simulink model "Exercise_3_1"  (R2022a)
settings: Solver=VariableStepAuto  StartTime=0.0  StopTime=30  RelTol=1e-3
libraries: simulink_extras x6, m3dof_library x6, simulink x2
settings Model: Creator=s9203  LastModifiedBy=s9203

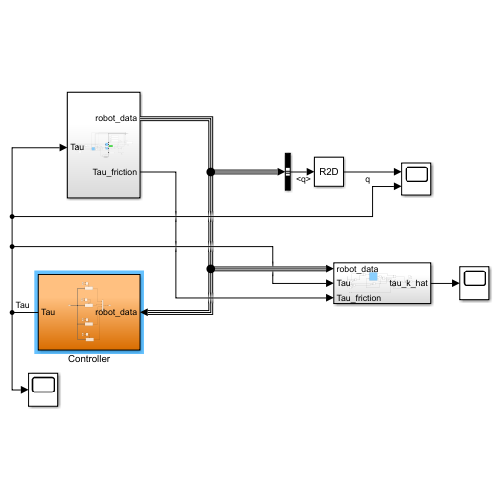
[thumbnail: Simulink's stored preview of the top-level diagram]
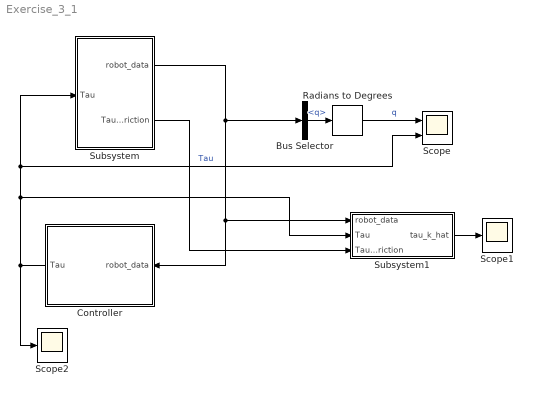
== system Exercise_3_1 ==
  Bus Selector : BusSelector  OutputSignals=q
  Controller : Subsystem
  Radians to Degrees : simulink_extras/Transformations/Radians to Degrees
  Scope : Scope  NumInputPorts=2
  Scope1 : Scope
  Scope2 : Scope
  Subsystem : Subsystem
  Subsystem1 : Subsystem
  wires:
  Subsystem/1(robot_data) -> Bus Selector/1, Controller/1(robot_data), Subsystem1/1(robot_data)
  Controller/1(Tau) -> Scope/2, Subsystem/1(Tau), Subsystem1/2(Tau), Scope2/1  "Tau"
  Bus Selector/1 -> Radians to Degrees/1  "<q>"
  Radians to Degrees/1 -> Scope/1  "q"
  Subsystem1/1(tau_k_hat) -> Scope1/1
  Subsystem/2(Tau_friction) -> Subsystem1/3(Tau_friction)

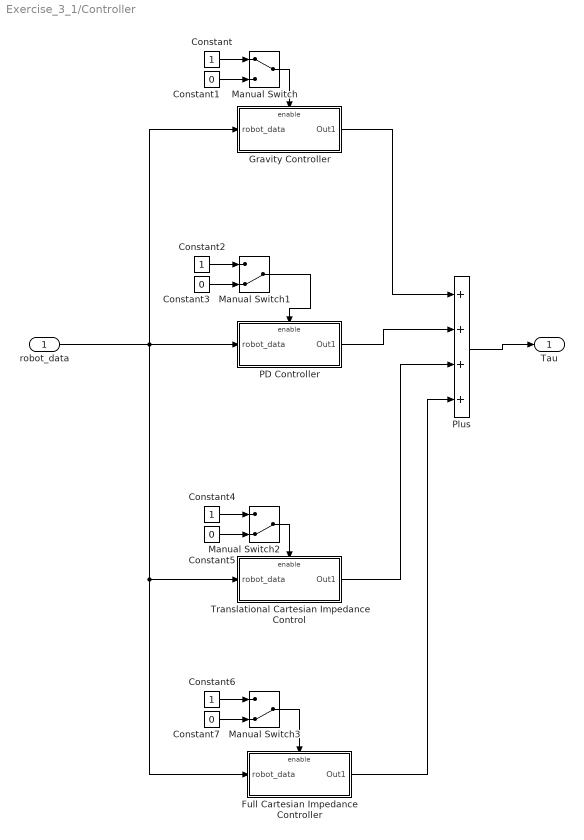
== system Exercise_3_1/Controller ==
  robot_data : Inport
  Constant{,2,4,6} (4 alike) : Constant
  Constant{1,3,5,7} (4 alike) : Constant  Value=0
  Full Cartesian Impedance Controller : Subsystem  TreatAsAtomicUnit=on
  Gravity Controller : Subsystem  TreatAsAtomicUnit=on
  Manual Switch : ManualSwitch
  Manual Switch1 : ManualSwitch  CurrentSetting=0
  Manual Switch2 : ManualSwitch  CurrentSetting=0
  Manual Switch3 : ManualSwitch  CurrentSetting=0
  "PD Controller " : Subsystem  TreatAsAtomicUnit=on
  Plus : Sum  Inputs=++++
  Translational Cartesian Impedance Control : Subsystem  TreatAsAtomicUnit=on
  Tau : Outport
  wires:
  robot_data/1 -> Full Cartesian Impedance Controller/1(robot_data), Translational Cartesian Impedance Control/1(robot_data), "PD Controller "/1(robot_data), Gravity Controller/1(robot_data)
  Gravity Controller/1(Out1) -> Plus/1
  "PD Controller "/1(Out1) -> Plus/2
  Translational Cartesian Impedance Control/1(Out1) -> Plus/3
  Plus/1 -> Tau/1
  Constant/1 -> Manual Switch/1
  Constant1/1 -> Manual Switch/2
  Manual Switch/1 -> Gravity Controller/Enable
  Constant3/1 -> Manual Switch1/2
  Constant2/1 -> Manual Switch1/1
  Constant4/1 -> Manual Switch2/1
  Constant5/1 -> Manual Switch2/2
  Manual Switch2/1 -> Translational Cartesian Impedance Control/Enable
  Manual Switch1/1 -> "PD Controller "/Enable
  Manual Switch3/1 -> Full Cartesian Impedance Controller/Enable
  Constant7/1 -> Manual Switch3/2
  Constant6/1 -> Manual Switch3/1
  Full Cartesian Impedance Controller/1(Out1) -> Plus/4

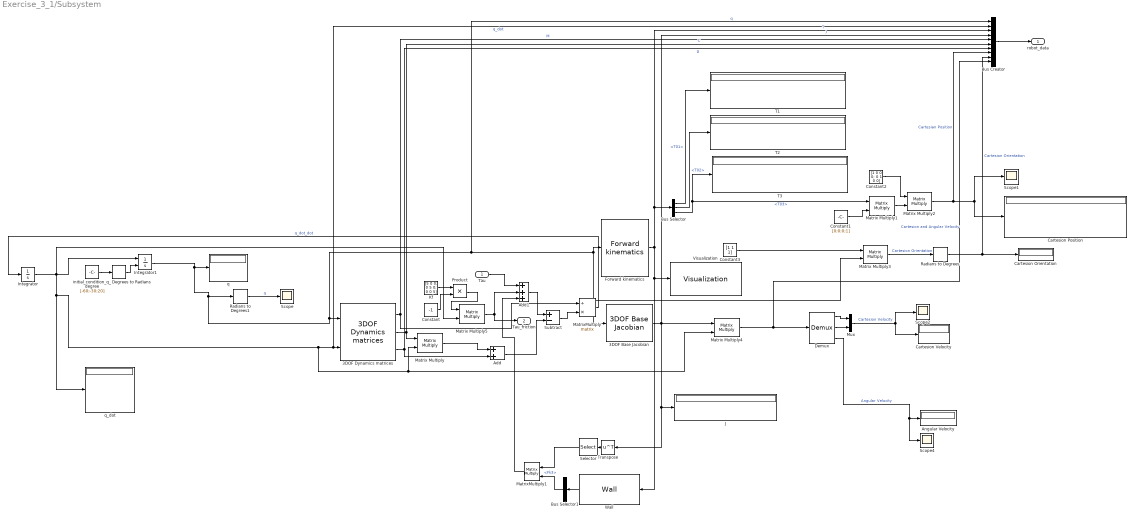
== system Exercise_3_1/Subsystem ==
  Tau : Inport
  3DOF Base Jacobian : m3dof_library/3DOF Base Jacobian  a1=l1  a2=l2  a3=l3
  3DOF Dynamics matrices : m3dof_library/3DOF Dynamics matrices  m1=m1  mX1=mx1  ZZ1=I1  m2=m2  mX2=mx2  ZZ2=I2  m3=m3  mX3=mx3  ZZ3=I3  a1=l1  a2=l2  a3=l3  eg=eg
  Add : Sum
  Add1 : Sum  Inputs=+++
  Angular Velocity : Display
  Bus Creator : BusCreator  Inputs=10
  Bus Selector : BusSelector  OutputSignals=T01,T02,T03
  Bus Selector1 : BusSelector  OutputSignals=Fk3
  Cartesion Orientation : Display
  Cartesion Position : Display
  Cartesion Velocity : Display
  Constant : Constant  Value=-1
  Constant1 : Constant  Value=[0;0;0;1]
  Constant2 : Constant  Value=[1 0 0 0; 0 1 0 0]
  Constant3 : Constant  Value=[1 1 1]  VectorParams1D=off
  Degrees to Radians : simulink_extras/Transformations/Degrees to Radians
  Demux : Demux  Outputs=3
      settings: DisplayOption=none
  Forward kinematics : m3dof_library/Forward kinematics  a1=l1  a2=l2  a3=l3  alpha=0
  Integrator : Integrator
  Integrator1 : Integrator  InitialConditionSource=external
  J : Display
  Kf : Constant  Value=[5 0 0; 0 5 0; 0 0 5]
  Matrix Multiply{,1..5} (6 alike) : Product  Multiplication=Matrix(*)
  MatrixMultiply : Product  Inputs=/*  Multiplication=Matrix(*)
  MatrixMultiply1 : Product  Multiplication=Matrix(*)
  Mux : Mux  Inputs=2
  Product : Product
  Radians to Degrees : simulink_extras/Transformations/Radians to Degrees
  Radians to Degrees1 : simulink_extras/Transformations/Radians to Degrees
  Scope{,1..2,4} (4 alike) : Scope
  Selector : Selector  NumberOfDimensions=2  InputPortWidth=3  IndexOptions=Index vector (dialog),Index vector (dialog)  Indices=[1 2 3],[1 2]  OutputSizes=1,1
  Subtract : Sum  Inputs=+-
  T1 : Display
  T2 : Display
  T3 : Display
  Transpose : Math  Operator=transpose
  Visualization : m3dof_library/Visualization  Ts0=1/16  al=1  a1=l1  a2=l2  a3=l3  alpha=0  eg=eg  tl=50
  Wall : m3dof_library/Wall  x0=[1.2 0]  w=[-1 0]
  "initial_condition_q_degree " : Constant  Value=[-60;-30;20]
  q : Display
  q_dot : Display
  robot_data : Outport
  Tau_friction : Outport  Port=2
  wires:
  Integrator/1 -> Matrix Multiply4/2, Matrix Multiply/2, Bus Creator/2, 3DOF Dynamics matrices/2, q_dot/1, Integrator1/1, Matrix Multiply5/2  "q_dot"
  Demux/3 -> Scope4/1, Angular Velocity/1  "Angular Velocity"
  3DOF Dynamics matrices/1 -> Bus Creator/5, MatrixMultiply/1  "M"
  Forward kinematics/1 -> Visualization/1, Wall/1, Bus Selector/1, Bus Creator/3  "T"
  Demux/1 -> Mux/1
  3DOF Base Jacobian/1 -> Transpose/1, J/1, Matrix Multiply4/1, Bus Creator/4  "J"
  Add1/1 -> Subtract/1
  Degrees to Radians/1 -> Integrator1/2
  Demux/2 -> Mux/2
  Matrix Multiply2/1 -> Bus Creator/8, Cartesion Position/1, Scope1/1  "Cartesian Position"
  3DOF Dynamics matrices/3 -> Bus Creator/7, Add/2  "g"
  Mux/1 -> Cartesion Velocity/1, Scope2/1  "Cartesion Velocity"
  Matrix Multiply/1 -> Add/1
  Radians to Degrees/1 -> Cartesion Orientation/1, Bus Creator/9  "Cartesion Orientation"
  MatrixMultiply/1 -> Integrator/1  "q_dot_dot"
  3DOF Dynamics matrices/2 -> Bus Creator/6, Matrix Multiply/1  "C"
  Constant/1 -> Product/2
  Matrix Multiply5/1 -> Add1/2, Tau_friction/1
  Bus Selector/3 -> Matrix Multiply1/1, T3/1  "<T03>"
  "initial_condition_q_degree "/1 -> Degrees to Radians/1
  Bus Selector/2 -> T2/1  "<T02>"
  Constant1/1 -> Matrix Multiply1/2
  Matrix Multiply3/1 -> Radians to Degrees/1  "Cartesion Orientation"
  Constant3/1 -> Matrix Multiply3/1
  Bus Selector/1 -> T1/1  "<T01>"
  Constant2/1 -> Matrix Multiply2/1
  Add/1 -> Subtract/2
  Matrix Multiply1/1 -> Matrix Multiply2/2
  Matrix Multiply4/1 -> Bus Creator/10, Demux/1  "Cartesion and Angular Velocity"
  Bus Creator/1 -> robot_data/1
  Kf/1 -> Product/1
  Product/1 -> Matrix Multiply5/1
  Integrator1/1 -> Radians to Degrees1/1, Bus Creator/1, 3DOF Base Jacobian/1, Matrix Multiply3/2, Forward kinematics/1, 3DOF Dynamics matrices/1, q/1  "q"
  Wall/1 -> Bus Selector1/1
  Transpose/1 -> Selector/1
  Selector/1 -> MatrixMultiply1/1
  Bus Selector1/1 -> MatrixMultiply1/2  "<Fk3>"
  MatrixMultiply1/1 -> Add1/3
  Subtract/1 -> MatrixMultiply/2
  Radians to Degrees1/1 -> Scope/1  "q"
  Tau/1 -> Add1/1

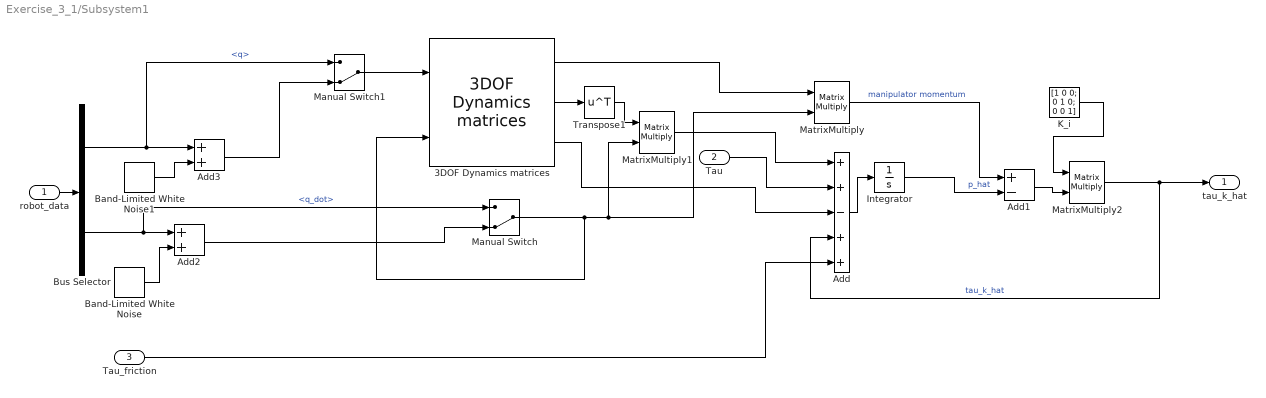
== system Exercise_3_1/Subsystem1 ==
  robot_data : Inport
  Tau : Inport  Port=2
  Tau_friction : Inport  Port=3
  3DOF Dynamics matrices : m3dof_library/3DOF Dynamics matrices  m1=m1  mX1=mx1  ZZ1=I1  m2=m2  mX2=mx2  ZZ2=I2  m3=m3  mX3=mx3  ZZ3=I3  a1=l1  a2=l2  a3=l3  eg=eg
  Add : Sum  Inputs=++-++
  Add1 : Sum  Inputs=+-
  Add2 : Sum
  Add3 : Sum
  Band-Limited White Noise : simulink/Sources/Band-Limited White Noise  Cov=[0.0001]  Ts=0.1  seed=[23341]
  Band-Limited White Noise1 : simulink/Sources/Band-Limited White Noise  Cov=[0.0001]  Ts=0.1  seed=[23341]
  Bus Selector : BusSelector  OutputSignals=q,q_dot
  Integrator : Integrator
  K_i : Constant  Value=[1 0 0; 0 1 0; 0 0 1]
  Manual Switch : ManualSwitch  CurrentSetting=0
  Manual Switch1 : ManualSwitch  CurrentSetting=0
  MatrixMultiply : Product  Multiplication=Matrix(*)
  MatrixMultiply1 : Product  Multiplication=Matrix(*)
  MatrixMultiply2 : Product  Multiplication=Matrix(*)
  Transpose1 : Math  Operator=transpose
  tau_k_hat : Outport
  wires:
  robot_data/1 -> Bus Selector/1
  3DOF Dynamics matrices/1 -> MatrixMultiply/1
  Manual Switch/1 -> MatrixMultiply/2, MatrixMultiply1/2, 3DOF Dynamics matrices/2
  3DOF Dynamics matrices/2 -> Transpose1/1
  Transpose1/1 -> MatrixMultiply1/1
  3DOF Dynamics matrices/3 -> Add/3
  Add/1 -> Integrator/1
  MatrixMultiply/1 -> Add1/1  "manipulator momentum"
  Integrator/1 -> Add1/2  "p_hat"
  Add1/1 -> MatrixMultiply2/2
  K_i/1 -> MatrixMultiply2/1
  MatrixMultiply2/1 -> Add/4, tau_k_hat/1  "tau_k_hat"
  Bus Selector/2 -> Manual Switch/1, Add2/1  "<q_dot>"
  Add2/1 -> Manual Switch/2
  Manual Switch1/1 -> 3DOF Dynamics matrices/1
  Bus Selector/1 -> Manual Switch1/1, Add3/1  "<q>"
  Add3/1 -> Manual Switch1/2
  Band-Limited White Noise1/1 -> Add3/2
  Band-Limited White Noise/1 -> Add2/2
  Tau/1 -> Add/2
  MatrixMultiply1/1 -> Add/1
  Tau_friction/1 -> Add/5

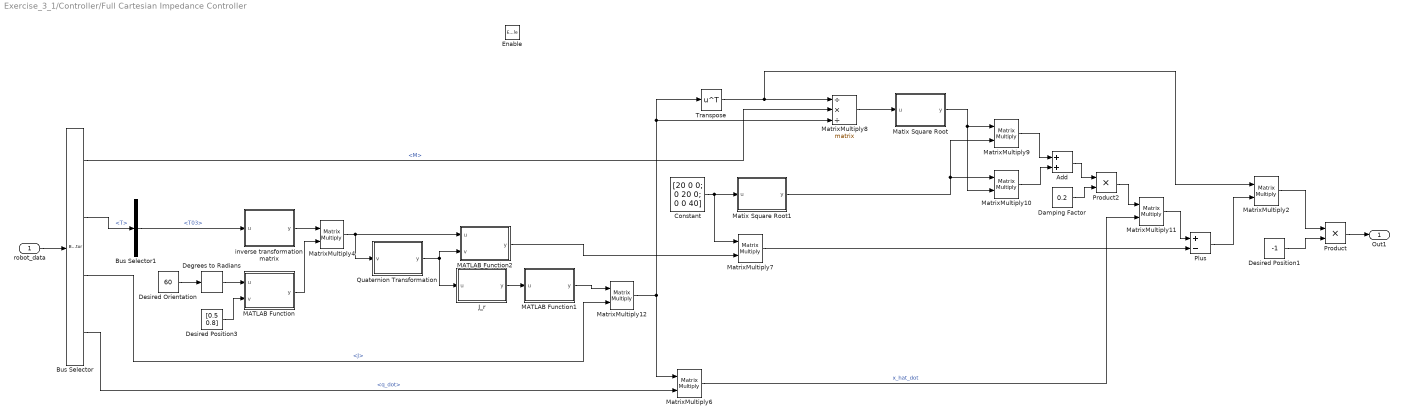
== system Exercise_3_1/Controller/Full Cartesian Impedance Controller ==
  robot_data : Inport
  Enable : EnablePort
  Add : Sum
  Bus Selector : BusSelector  OutputSignals=M,T,J,q_dot
  Bus Selector1 : BusSelector  OutputSignals=T03
  Constant : Constant  Value=[20 0 0; 0 20 0; 0 0 40]  VectorParams1D=off
  Damping Factor : Constant  Value=0.2
  Degrees to Radians : simulink_extras/Transformations/Degrees to Radians
  Desired Orientation : Constant  Value=60
  Desired Position1 : Constant  Value=-1
  Desired Position3 : Constant  Value=[0.5 0.8]  VectorParams1D=off
  J_r : MATLAB Function  TreatAsAtomicUnit=on
  MATLAB Function : MATLAB Function  TreatAsAtomicUnit=on
  MATLAB Function1 : MATLAB Function  TreatAsAtomicUnit=on
  MATLAB Function2 : MATLAB Function  TreatAsAtomicUnit=on
  Matix Square Root : MATLAB Function  TreatAsAtomicUnit=on
  Matix Square Root1 : MATLAB Function  TreatAsAtomicUnit=on
  MatrixMultiply{2,4,6..7,9..12} (8 alike) : Product  Multiplication=Matrix(*)
  MatrixMultiply8 : Product  Inputs=/*/  Multiplication=Matrix(*)
  Plus : Sum  Inputs=+-
  Product : Product
  Product2 : Product
  Quaternion Transformation : MATLAB Function  TreatAsAtomicUnit=on
  Transpose : Math  Operator=transpose
  inverse transformation matrix : MATLAB Function  TreatAsAtomicUnit=on
  Out1 : Outport
  wires:
  Transpose/1 -> MatrixMultiply2/1, MatrixMultiply8/1
  Desired Position1/1 -> Product/2
  MatrixMultiply2/1 -> Product/1
  Bus Selector/3 -> MatrixMultiply12/2  "<J>"
  Desired Position3/1 -> MATLAB Function/2(v)
  robot_data/1 -> Bus Selector/1
  Bus Selector/2 -> Bus Selector1/1  "<T>"
  Bus Selector1/1 -> inverse transformation matrix/1(u)  "<T03>"
  J_r/1(y) -> MATLAB Function1/1(u)
  Desired Orientation/1 -> Degrees to Radians/1
  Degrees to Radians/1 -> MATLAB Function/1(u)
  Bus Selector/4 -> MatrixMultiply6/2  "<q_dot>"
  MATLAB Function1/1(y) -> MatrixMultiply12/1
  MatrixMultiply6/1 -> MatrixMultiply11/2  "x_hat_dot"
  Quaternion Transformation/1(y) -> J_r/1(u), MATLAB Function2/2(v)
  Constant/1 -> MatrixMultiply7/1, Matix Square Root1/1(u)
  Bus Selector/1 -> MatrixMultiply8/2  "<M>"
  MatrixMultiply8/1 -> Matix Square Root/1(u)
  Matix Square Root/1(y) -> MatrixMultiply10/2, MatrixMultiply9/1
  Matix Square Root1/1(y) -> MatrixMultiply9/2, MatrixMultiply10/1
  MatrixMultiply9/1 -> Add/1
  MatrixMultiply10/1 -> Add/2
  Add/1 -> Product2/1
  Damping Factor/1 -> Product2/2
  Product2/1 -> MatrixMultiply11/1
  MatrixMultiply12/1 -> MatrixMultiply8/3, Transpose/1, MatrixMultiply6/1
  MATLAB Function/1(y) -> MatrixMultiply4/2
  inverse transformation matrix/1(y) -> MatrixMultiply4/1
  MatrixMultiply4/1 -> Quaternion Transformation/1(v), MATLAB Function2/1(u)
  Product/1 -> Out1/1
  MatrixMultiply7/1 -> Plus/2
  MatrixMultiply11/1 -> Plus/1
  Plus/1 -> MatrixMultiply2/2
  MATLAB Function2/1(y) -> MatrixMultiply7/2

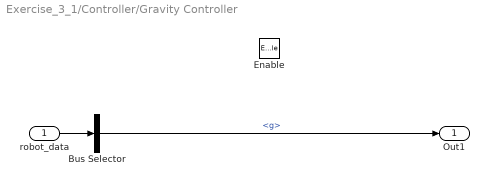
== system Exercise_3_1/Controller/Gravity Controller ==
  robot_data : Inport
  Enable : EnablePort
  Bus Selector : BusSelector  OutputSignals=g
  Out1 : Outport
  wires:
  robot_data/1 -> Bus Selector/1
  Bus Selector/1 -> Out1/1  "<g>"

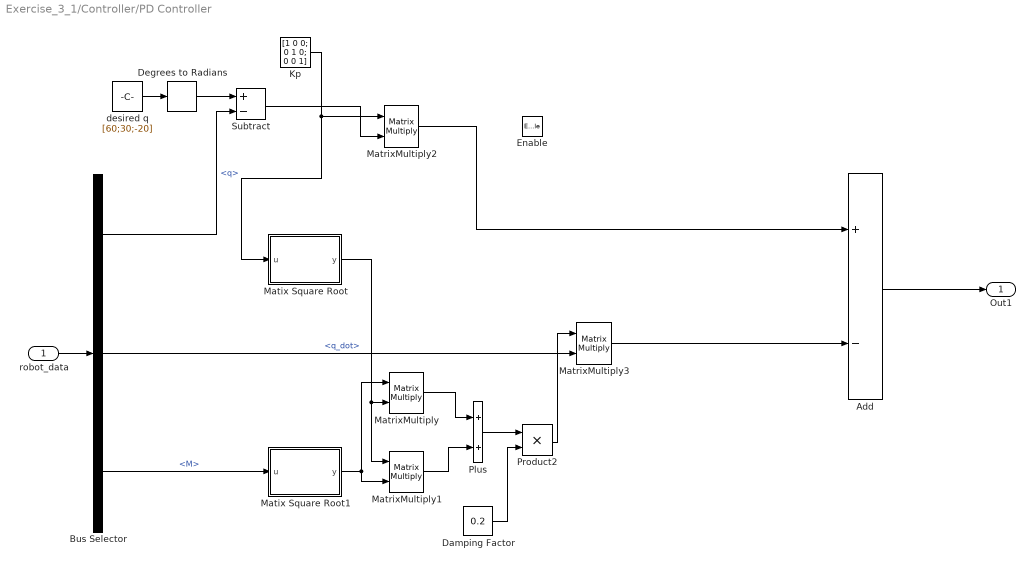
== system Exercise_3_1/Controller/PD Controller  ==
  robot_data : Inport
  Enable : EnablePort
  Add : Sum  Inputs=+-
  Bus Selector : BusSelector  OutputSignals=q,q_dot,M
  Damping Factor : Constant  Value=0.2
  Degrees to Radians : simulink_extras/Transformations/Degrees to Radians
  Kp : Constant  Value=[1 0 0; 0 1 0; 0 0 1]
  Matix Square Root : MATLAB Function  TreatAsAtomicUnit=on
  Matix Square Root1 : MATLAB Function  TreatAsAtomicUnit=on
  MatrixMultiply{,1..3} (4 alike) : Product  Multiplication=Matrix(*)
  Plus : Sum
  Product2 : Product
  Subtract : Sum  Inputs=+-
  desired q : Constant  Value=[60;30;-20]
  Out1 : Outport
  wires:
  Add/1 -> Out1/1
  desired q/1 -> Degrees to Radians/1
  robot_data/1 -> Bus Selector/1
  Degrees to Radians/1 -> Subtract/1
  Bus Selector/1 -> Subtract/2  "<q>"
  Subtract/1 -> MatrixMultiply2/2
  Kp/1 -> Matix Square Root/1(u), MatrixMultiply2/1
  MatrixMultiply2/1 -> Add/1
  MatrixMultiply3/1 -> Add/2
  Bus Selector/2 -> MatrixMultiply3/2  "<q_dot>"
  Bus Selector/3 -> Matix Square Root1/1(u)  "<M>"
  Matix Square Root1/1(y) -> MatrixMultiply1/2, MatrixMultiply/1
  Matix Square Root/1(y) -> MatrixMultiply1/1, MatrixMultiply/2
  MatrixMultiply/1 -> Plus/1
  MatrixMultiply1/1 -> Plus/2
  Plus/1 -> Product2/1
  Damping Factor/1 -> Product2/2
  Product2/1 -> MatrixMultiply3/1

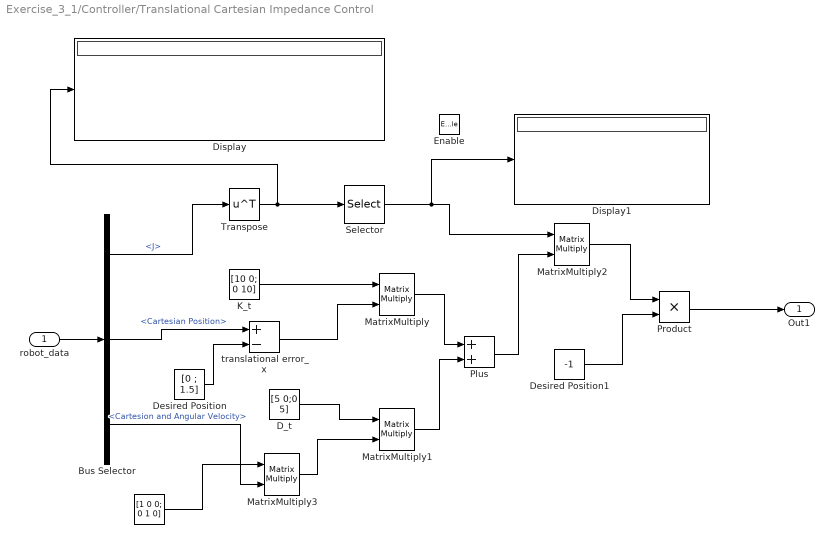
== system Exercise_3_1/Controller/Translational Cartesian Impedance Control ==
  robot_data : Inport
  Enable : EnablePort
  " " : Constant  Value=[1 0 0; 0 1 0]
  Bus Selector : BusSelector  OutputSignals=J,Cartesian Position,Cartesion and Angular Velocity
  D_t : Constant  Value=[5 0;0 5]
  Desired Position : Constant  Value=[0 ; 1.5]
  Desired Position1 : Constant  Value=-1
  Display : Display
  Display1 : Display
  K_t : Constant  Value=[10 0; 0 10]
  MatrixMultiply{,1..3} (4 alike) : Product  Multiplication=Matrix(*)
  Plus : Sum
  Product : Product
  Selector : Selector  NumberOfDimensions=2  InputPortWidth=3  IndexOptions=Index vector (dialog),Index vector (dialog)  Indices=[1 2 3],[1 2]  OutputSizes=1,1
  Transpose : Math  Operator=transpose
  translational error_x : Sum  Inputs=+-
  Out1 : Outport
  wires:
  robot_data/1 -> Bus Selector/1
  Desired Position/1 -> translational error_x/2
  Bus Selector/2 -> translational error_x/1  "<Cartesian Position>"
  K_t/1 -> MatrixMultiply/1
  translational error_x/1 -> MatrixMultiply/2
  D_t/1 -> MatrixMultiply1/1
  Bus Selector/1 -> Transpose/1  "<J>"
  MatrixMultiply/1 -> Plus/1
  MatrixMultiply1/1 -> Plus/2
  Plus/1 -> MatrixMultiply2/2
  MatrixMultiply2/1 -> Product/1
  Desired Position1/1 -> Product/2
  Product/1 -> Out1/1
  " "/1 -> MatrixMultiply3/1
  Bus Selector/3 -> MatrixMultiply3/2  "<Cartesion and Angular Velocity>"
  MatrixMultiply3/1 -> MatrixMultiply1/2
  Transpose/1 -> Display/1, Selector/1
  Selector/1 -> Display1/1, MatrixMultiply2/1

== matlab function Exercise_3_1/Controller/PD Controller /Matix Square Root1 ==
  data: u input; y output
function y = fcn(u)

y = real(sqrtm(u));

== matlab function Exercise_3_1/Controller/PD Controller /Matix Square Root ==
  data: u input; y output
function y = fcn(u)

y = real(sqrtm(u));

== matlab function Exercise_3_1/Controller/Full Cartesian Impedance Controller/J_r ==
  data: u input; y output
function y = fcn(u)
eta= u(1,1);
diag_eta = eta*[1 0 0; 0 1 0; 0 0 1];

epsilon = [-u(2,1) -u(3,1) -u(4,1)]';
skew_epsilon = [0 -epsilon(3) epsilon(2) ; epsilon(3) 0 -epsilon(1) ; -epsilon(2) epsilon(1) 0 ];

y = skew_epsilon + diag_eta;

== matlab function Exercise_3_1/Controller/Full Cartesian Impedance Controller/Quaternion Transformation ==
  data: v input; y output
function y = fcn(v)
u = v(1:3,1:3);

eta = 0.5*sqrt([1 1 1]*(diag(u).^2)+1);

epsilon_1 = (u(3,2)-u(2,3))/(4*eta);
epsilon_2 = (u(1,3)-u(3,1))/(4*eta);
epsilon_3 = (u(2,1)-u(1,2))/(4*eta);

y = [eta ; epsilon_1; epsilon_2; epsilon_3];

== matlab function Exercise_3_1/Controller/Full Cartesian Impedance Controller/MATLAB Function ==
  data: u input; y output; v input
function y = fcn(u,v)
Transformation_matrix = [cos(u) -sin(u) 0 v(1); sin(u) cos(u) 0 v(2); 0 0 1 0; 0 0 0 1];

y = Transformation_matrix;

== matlab function Exercise_3_1/Controller/Full Cartesian Impedance Controller/MATLAB Function1 ==
  data: u input; y output
function y = fcn(u)


y = [1 0 0; 0 1 0; 0 0 u(3,3)];

== matlab function Exercise_3_1/Controller/Full Cartesian Impedance Controller/Matix Square Root ==
  data: u input; y output
function y = fcn(u)

y = real(sqrtm(u));

== matlab function Exercise_3_1/Controller/Full Cartesian Impedance Controller/Matix Square Root1 ==
  data: u input; y output
function y = fcn(u)

y = real(sqrtm(u));

== matlab function Exercise_3_1/Controller/Full Cartesian Impedance Controller/inverse transformation matrix ==
  data: u input; y output
function y = fcn(u)

R = u(1:3,1:3);

p = u(1:3,4);

T_tcp0 = [transpose(R) -transpose(R)*p; 0 0 0 1];


y = T_tcp0;

== matlab function Exercise_3_1/Controller/Full Cartesian Impedance Controller/MATLAB Function2 ==
  data: u input; y output; v input
function y = fcn(u,v)

y = [u(1:2,4); 2*v(4)];
